simulink model "Factoral"  (R2016b)
settings: Solver=FixedStepDiscrete  StartTime=0.0  StopTime=10.0  FixedStep=0.1  RelTol=1e-3  EnableMultiTasking=on
settings Model: Creator=Saher Ghanem  LastModifiedBy=Saher Ghanem
settings SolverCC: AutoInsertRateTranBlk=on
settings DataIOCC: LimitDataPoints=on
settings OptimizationCC: LifeSpan=inf
settings DebuggingCC: AllowSymbolicDim=off  SFUnexpectedBacktrackingDiag=warning  SFNoUnconditionalDefaultTransitionDiag=warning  SFExecutionAtInitializationDiag=none
settings GRTTargetCC: TargetLangStandard=C89/C90 (ANSI)  GeneratePreprocessorConditionals=Disable all
settings ConfigComp: CovMetricSettings=dw  CovHtmlReporting=on  CovSaveCumulativeToWorkspaceVar=on  CovSaveSingleToWorkspaceVar=on  CovExternalEMLEnable=off  CovSFcnEnable=off

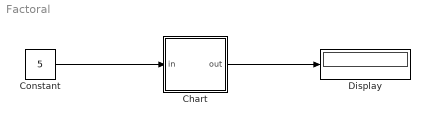
== system Factoral ==
  Chart : Stateflow chart  TreatAsAtomicUnit=on
  Constant : Constant  Value=5
  Display : Display
  wires:
  Constant/1 -> Chart/1(in)
  Chart/1(out) -> Display/1

== stateflow chart Factoral/Chart ==
  (default) -> (junction 10) : % Factorial
  (junction 10) -> (junction 12) : {var=in; res=1;}
  (junction 12) -> (junction 11) [order 1] : [var>0]
  (junction 11) -> (junction 13) : {res=var*res; var=var-1;}
  (junction 13) -> (junction 12)
  (junction 12) -> (junction 14) [order 2] : {out=res;}
  data: in input; out output =1; var local; res local
